simulink model "hgo_diff_new_ibrir"  (R2024b)
settings: Solver=FixedStepAuto  StartTime=0.0  StopTime=15  FixedStep=1e-5  RelTol=1e-3
libraries: simulink x1
settings Model: Creator=user  LastModifiedBy=user

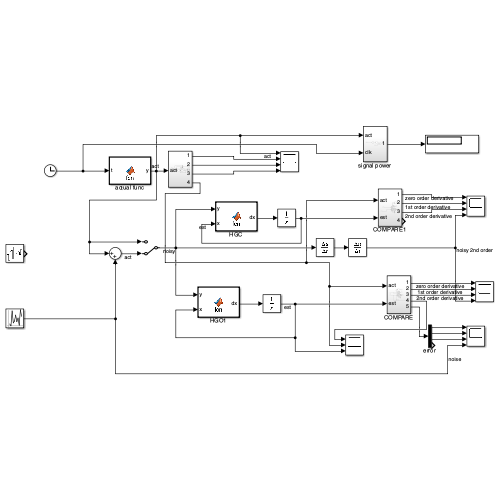
[thumbnail: Simulink's stored preview of the top-level diagram]
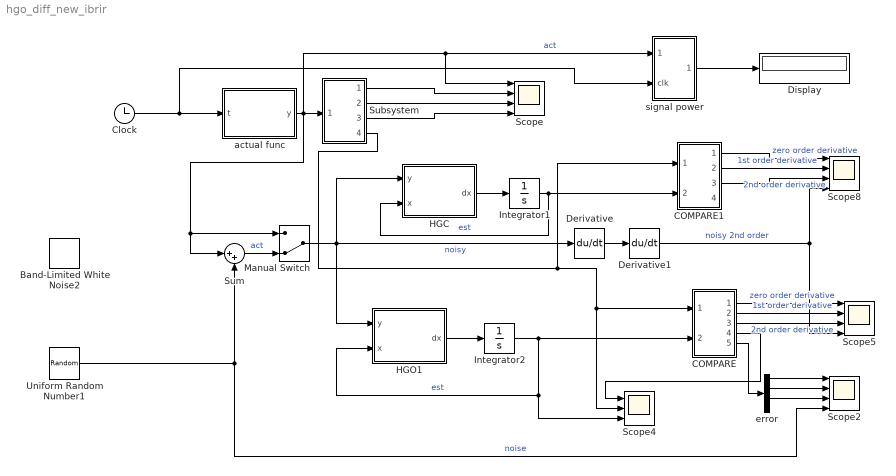
== system hgo_diff_new_ibrir ==
  Band-Limited White Noise2 : simulink/Sources/Band-Limited White Noise  Cov=1e-8  Ts=0.001  seed=[23341]
  COMPARE : Subsystem
  COMPARE1 : Subsystem
  Clock : Clock
  Derivative : Derivative
  Derivative1 : Derivative
  Display : Display
  HGC : MATLAB Function  TreatAsAtomicUnit=on
  HGO1 : MATLAB Function  TreatAsAtomicUnit=on
  Integrator1 : Integrator
  Integrator2 : Integrator
  Manual Switch : ManualSwitch  CurrentSetting=0
  Scope{,2,5,8} (4 alike) : Scope  NumInputPorts=4
  Scope4 : Scope  NumInputPorts=3
  Subsystem : Subsystem
  Sum : Sum  Inputs=|++
  Uniform Random Number1 : UniformRandomNumber  Minimum=-1e-3  Maximum=1e-3  SampleTime=1e-3
  actual func : MATLAB Function  TreatAsAtomicUnit=on
  error : Demux
  signal power : Subsystem
  wires:
  actual func/1(y) -> Manual Switch/1, Sum/1, Subsystem/1(act), signal power/1(act), Scope/1  "act"
  HGC/1(dx) -> Integrator1/1
  Integrator1/1 -> COMPARE1/2(est), HGC/2(x)  "est"
  Sum/1 -> Manual Switch/2  "act"
  Manual Switch/1 -> Derivative/1, HGC/1(y), HGO1/1(y)  "noisy"
  HGO1/1(dx) -> Integrator2/1
  Integrator2/1 -> COMPARE/2(est), Scope4/3, HGO1/2(x)  "est"
  Clock/1 -> actual func/1(t), signal power/2(clk)
  COMPARE/1(Out1) -> Scope5/1  "zero order derivative"
  COMPARE/2(Out2) -> Scope5/2  "1st order derivative"
  COMPARE/3(Out3) -> Scope5/3  "2nd order derivative"
  Subsystem/4(Out4) -> Scope4/2, COMPARE/1(act), COMPARE1/1(act)
  Subsystem/1(Out1) -> Scope/2
  Subsystem/2(Out2) -> Scope/3
  Subsystem/3(Out3) -> Scope/4
  COMPARE1/1(Out1) -> Scope8/1  "zero order derivative"
  COMPARE1/2(Out2) -> Scope8/2  "1st order derivative"
  COMPARE1/3(Out3) -> Scope8/3  "2nd order derivative"
  Derivative/1 -> Derivative1/1
  Derivative1/1 -> Scope5/4, Scope8/4  "noisy 2nd order"
  Uniform Random Number1/1 -> Sum/2, Scope2/4  "noise"
  signal power/1(Out1) -> Display/1
  COMPARE/4(Out4) -> Scope4/1
  COMPARE/5(Out5) -> error/1
  error/1 -> Scope2/1
  error/2 -> Scope2/2
  error/3 -> Scope2/3

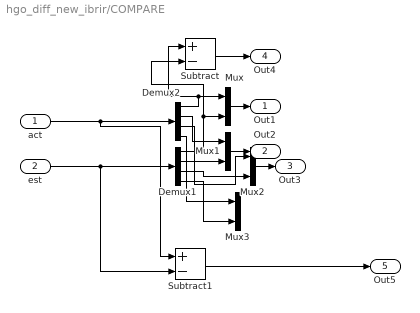
== system hgo_diff_new_ibrir/COMPARE ==
  act : Inport
  est : Inport  Port=2
  Demux1 : Demux
  Demux2 : Demux
  Mux{,1..3} (4 alike) : Mux  Inputs=2
  Subtract : Sum  Inputs=+-
  Subtract1 : Sum  Inputs=+-
  Out1 : Outport
  Out2 : Outport  Port=2
  Out3 : Outport  Port=3
  Out4 : Outport  Port=4
  Out5 : Outport  Port=5
  wires:
  est/1 -> Subtract1/2, Demux1/1
  Demux1/3 -> Mux2/2
  act/1 -> Subtract1/1, Demux2/1
  Demux2/1 -> Subtract/1, Mux/1
  Mux/1 -> Out1/1
  Demux1/2 -> Mux1/2
  Demux1/1 -> Subtract/2, Mux/2
  Demux2/2 -> Mux1/1
  Mux2/1 -> Out3/1
  Demux2/3 -> Mux2/1
  Demux2/4 -> Mux3/1
  Mux1/1 -> Out2/1
  Demux1/4 -> Mux3/2
  Subtract/1 -> Out4/1
  Subtract1/1 -> Out5/1

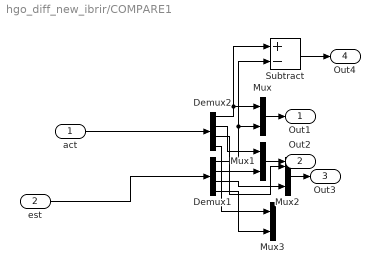
== system hgo_diff_new_ibrir/COMPARE1 ==
  act : Inport
  est : Inport  Port=2
  Demux1 : Demux
  Demux2 : Demux
  Mux{,1..3} (4 alike) : Mux  Inputs=2
  Subtract : Sum  Inputs=+-
  Out1 : Outport
  Out2 : Outport  Port=2
  Out3 : Outport  Port=3
  Out4 : Outport  Port=4
  wires:
  Demux1/4 -> Mux3/2
  Mux1/1 -> Out2/1
  Demux2/4 -> Mux3/1
  Demux2/3 -> Mux2/1
  Mux2/1 -> Out3/1
  Demux2/2 -> Mux1/1
  Demux1/1 -> Subtract/2, Mux/2
  Demux1/2 -> Mux1/2
  Mux/1 -> Out1/1
  Demux2/1 -> Subtract/1, Mux/1
  act/1 -> Demux2/1
  Demux1/3 -> Mux2/2
  est/1 -> Demux1/1
  Subtract/1 -> Out4/1

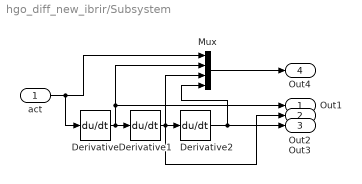
== system hgo_diff_new_ibrir/Subsystem ==
  act : Inport
  Derivative : Derivative
  Derivative1 : Derivative
  Derivative2 : Derivative
  Mux : Mux
  Out1 : Outport
  Out2 : Outport  Port=2
  Out3 : Outport  Port=3
  Out4 : Outport  Port=4
  wires:
  Derivative/1 -> Out1/1, Mux/2, Derivative1/1
  Derivative1/1 -> Out2/1, Mux/3, Derivative2/1
  act/1 -> Derivative/1, Mux/1
  Mux/1 -> Out4/1
  Derivative2/1 -> Out3/1, Mux/4

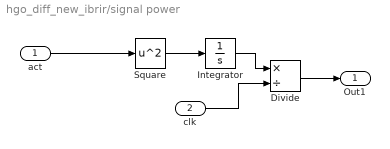
== system hgo_diff_new_ibrir/signal power ==
  act : Inport
  clk : Inport  Port=2
  Divide : Product  Inputs=*/
  Integrator : Integrator
  Square : Math  Operator=square
  Out1 : Outport
  wires:
  Square/1 -> Integrator/1
  act/1 -> Square/1
  Integrator/1 -> Divide/1
  clk/1 -> Divide/2
  Divide/1 -> Out1/1

== matlab function hgo_diff_new_ibrir/HGC ==
  data: y input; dx output; x input
function dx = fcn(y, x)
 
    %   dx_i = x_{i+1},   for 1 ≤ i ≤ n-1
    %   dx_n = -(mu*t)^n * (x_1 - y) - sum( C(n, i) * (mu*t)^i * x_{n-i+1} )

    n = 4;
    mu = 90; % hgo gain 
    %t = t/5; % scaling factor compromise between peak and accuracy
    %a = 1; 
    t = 1;

    % Ci = nchoosek(n, i)
    C = [4, 6, 4, 1];

    % Initialize derivative vector
    dx = zeros(n, 1);

    % First three equations: dx_i = x_{i+1}
    dx(1) = x(2);
    dx(2) = x(3);
    dx(3) = x(4);

    % Compute dx_4 using the given formula
    dx(4) = - (mu*t)^4 * (x(1) - y) - (C(1)*(mu*t)^1*x(4)) ... 
            - (C(2)*(mu*t)^2* x(3)) - (C(3)*(mu*t)^3*x(2));
end

== matlab function hgo_diff_new_ibrir/actual func ==
  data: t input; y output
function y = fcn(t)
%y = -(1 + exp(-2*t)) * sin(2*t)/(5 + cos(t));
y = -cos(t)/(2+sin(3*t));
% y = sin(t) + cos(5*t);
% dy = cos(t) - 5*sin(5*t);
% d2y = -sin(t) - 25*cos(5*t);
% d3y = -cos(t) + 125*sin(5*t);
% d4y = sin(t) + 625*cos(5*t);

% yt = [y; dy; d2y; d3y];

== matlab function hgo_diff_new_ibrir/HGO1 ==
  data: y input; dx output; x input
function dx = fcn(y, x)
    % Parameters
    n = 4;                % Order of the observer
    epsilon = 1/50;      % Small gain parameter
    % tr = 1 ; 
    % Binomial coefficients (for n = 4)
    % ki = nchoosek(n, i)
    k = [4, 6, 4, 1]; 

    % Initialize output derivative
    dx = zeros(n, 1);
    
    % High-Gain Observer Equations
    dx(1) = x(2) + (k(1) / epsilon^1) * (y - x(1));
    dx(2) = x(3) + (k(2) / epsilon^2) * (y - x(1));
    dx(3) = x(4) + (k(3) / epsilon^3) * (y - x(1));
    dx(4) = (k(4) / epsilon^4) * (y - x(1));
end
